simulink model "bsm1_ss_settlerreactive_standalone"  (Simulink 8.0)
settings: Solver=ode15s  SolverMode=SingleTasking  StartTime=0.0  StopTime=200  FixedStep=0.01  RelTol=1e-5  AbsTol=1e-8
undefined symbols (not defined in the file or in its folder): Qr, Qw
settings Model: Creator=ielulf  LastModifiedBy=lasn  ExtModeTrigMode=oneshot  ExtModeArmWhenConnect=off  ExtModeAutoUpdateStatusClock=off  BufferReuse=off
settings DataIOCC: InitialState=xFinal  LimitDataPoints=off  SignalLoggingSaveFormat=ModelDataLogs  SaveOutput=off  TimeSaveName=t  SignalLoggingName=sigsOut  OutputTimes=[0:(1/96):609]
settings OptimizationCC: BlockReduction=off  BooleanDataType=off  InlineInvariantSignals=on  OptimizeBlockIOStorage=off  BufferReuse=off  ExpressionFolding=off  LocalBlockOutputs=off  InitFltsAndDblsToZero=on
settings DebuggingCC: SaveWithParameterizedLinksMsg=none  SignalResolutionControl=TryResolveAllWithWarning  SolverPrmCheckMsg=none  InheritedTsInSrcMsg=none  MultiTaskDSMMsg=warning  MultiTaskCondExecSysMsg=none  FcnCallInpInsideContextMsg=UseLocalSettings  UnconnectedOutputMsg=none  StrictBusMsg=None
settings HardwareCC: TargetUnknown=on
settings RTWCC: TemplateMakefile=grt_unix.tmf  IncludeERTFirstTime=on
settings GRTTargetCC: TargetFcnLib=ansi_tfl_tmw.mat  CombineOutputUpdateFcns=off  GRTInterface=on

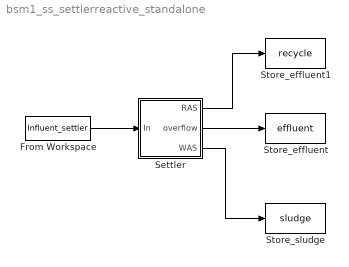
== system bsm1_ss_settlerreactive_standalone ==
  From Workspace : FromWorkspace  VariableName=Influent_settler
  Settler : Subsystem
  Store_effluent : ToWorkspace  VariableName=effluent
  Store_effluent1 : ToWorkspace  VariableName=recycle
  Store_sludge : ToWorkspace  VariableName=sludge
  wires:
  Settler/2(overflow) -> Store_effluent/1
  Settler/3(WAS) -> Store_sludge/1
  Settler/1(RAS) -> Store_effluent1/1
  From Workspace/1 -> Settler/1(In)

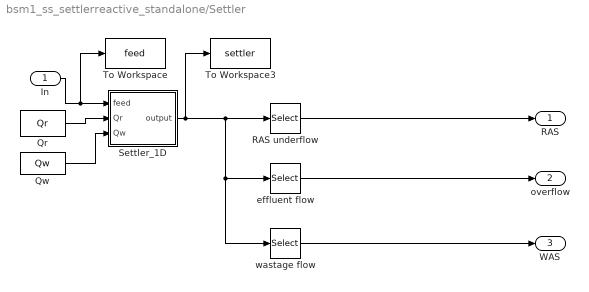
== system bsm1_ss_settlerreactive_standalone/Settler ==
  In : Inport
  Qr : Constant  Value=Qr
  Qw : Constant  Value=Qw
  RAS underflow : Selector  InputPortWidth=253  IndexOptions=Index vector (dialog)  Indices=[226 227 228 229 230 231 232 233 234 235 236 237 238 239 252 240 241 242 243 244 245 246 247 248 249 250]  OutputSizes=1
  Settler_1D : Subsystem
  To Workspace : ToWorkspace  VariableName=feed
  To Workspace3 : ToWorkspace  VariableName=settler
  effluent flow : Selector  InputPortWidth=253  IndexOptions=Index vector (dialog)  Indices=[1:14, 251, 15:25]  OutputSizes=1
  wastage flow : Selector  InputPortWidth=253  IndexOptions=Index vector (dialog)  Indices=[226:239, 253, 240:250]  OutputSizes=1
  RAS : Outport
  overflow : Outport  Port=2
  WAS : Outport  Port=3
  wires:
  In/1 -> To Workspace/1, Settler_1D/1(feed)
  Settler_1D/1(output) -> RAS underflow/1, effluent flow/1, wastage flow/1, To Workspace3/1
  wastage flow/1 -> WAS/1
  effluent flow/1 -> overflow/1
  RAS underflow/1 -> RAS/1
  Qr/1 -> Settler_1D/2(Qr)
  Qw/1 -> Settler_1D/3(Qw)

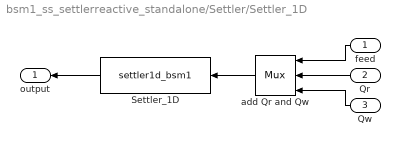
== system bsm1_ss_settlerreactive_standalone/Settler/Settler_1D ==
  feed : Inport
  Qr : Inport  Port=2
  Qw : Inport  Port=3
  Settler_1D : S-Function  FunctionName=settler1d_bsm1  Parameters=SETTLERINIT,SETTLERPAR,DIM,LAYER,TEMPMODEL, ACTIVATE  EnableBusSupport=off
  add Qr and Qw : Mux  Inputs=3
  output : Outport
  wires:
  Settler_1D/1 -> output/1
  feed/1 -> add Qr and Qw/1
  Qw/1 -> add Qr and Qw/3
  Qr/1 -> add Qr and Qw/2
  add Qr and Qw/1 -> Settler_1D/1
